simulink library "JointLib"  (R2021a)
settings: Solver=VariableStepAuto  StartTime=0.0  StopTime=10.0  RelTol=1e-3
values from neighbouring files (symbols this model uses):
  clientID = vrep.simxStart('127.0.0.1', port, true, true, 5000, 5)    [InitSim.m]
  vrep = remApi('remoteApi')    [InitSim.m]
settings Model: Creator=Harry  LastModifiedBy=Harry

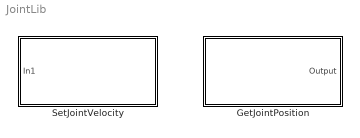
== system JointLib ==
  GetJointPosition : Subsystem  mask{joint_name='Revolute_joint1', is_use_radian=off}
      mask prompts: joint_name "Joint name"; is_use_radian "Is use radian"
      mask DialogControl DescGroupVar Prompt: Instructions
      mask DialogControl DescTextVar Prompt: ......
      mask Display:
      | if ischar(joint_name)
      |     color('black');
      |     x=sprintf('GetJointPosition\n%s',joint_name);
      |     disp(x);
      | else
      |     color('red');
      |     disp('Input Error');
      | end
  SetJointVelocity : Subsystem  mask{joint_name='Revolute_joint1', is_use_radian=on}
      mask prompts: joint_name "Joint name"; is_use_radian "Is use radian"
      mask DialogControl DescGroupVar Prompt: Instructions
      mask DialogControl DescTextVar Prompt: ......
      mask Display:
      | if ischar(joint_name)
      |     color('black');
      |     x=sprintf('SetJointVelocity\n%s',joint_name);
      |     disp(x);
      | else
      |     color('red');
      |     disp('Input Error');
      | end

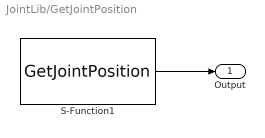
== system JointLib/GetJointPosition ==
  S-Function1 : S-Function  FunctionName=GetJointPosition  Parameters=vrep,clientID,joint_name,is_use_radian  SFunctionDeploymentMode=off  EnableBusSupport=off
  Output : Outport
  wires:
  S-Function1/1 -> Output/1

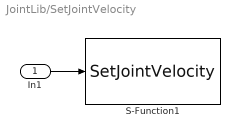
== system JointLib/SetJointVelocity ==
  In1 : Inport
  S-Function1 : S-Function  FunctionName=SetJointVelocity  Parameters=vrep,clientID,joint_name,is_use_radian  SFunctionDeploymentMode=off  EnableBusSupport=off
  wires:
  In1/1 -> S-Function1/1
